simulink model "flow_control_while"  (R2013b)
settings: Solver=ode45  StartTime=0.0  StopTime=10.0  RelTol=1e-3
libraries: simulink x2
settings Model: Creator=Administrator  LastModifiedBy=Administrator

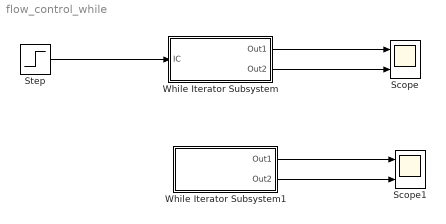
== system flow_control_while ==
  Scope : Scope  NumInputPorts=2
      settings: YMin=-5~-5  YMax=5~5
  Scope1 : Scope  NumInputPorts=2
      settings: YMin=-5~-5  YMax=5~5
  Step : Step  Time=5  SampleTime=0
  While Iterator Subsystem : Subsystem  TreatAsAtomicUnit=on
  While Iterator Subsystem1 : Subsystem  TreatAsAtomicUnit=on
  wires:
  Step/1 -> While Iterator Subsystem/1(IC)
  While Iterator Subsystem/1(Out1) -> Scope/1
  While Iterator Subsystem/2(Out2) -> Scope/2
  While Iterator Subsystem1/1(Out1) -> Scope1/1
  While Iterator Subsystem1/2(Out2) -> Scope1/2

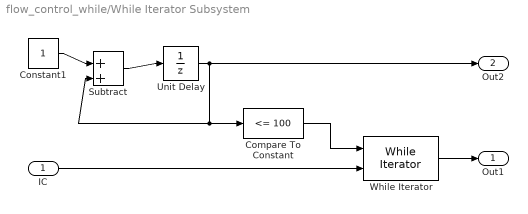
== system flow_control_while/While Iterator Subsystem ==
  IC : Inport
  Compare To Constant : simulink/Logic and Bit Operations/Compare To Constant  relop=<=  const=100  OutDataTypeStr=boolean
  Constant1 : Constant
  Subtract : Sum  Inputs=+|+
  Unit Delay : UnitDelay  SampleTime=-1
  While Iterator : WhileIterator  ShowIterationPort=on  OutputDataType=double
  Out1 : Outport
  Out2 : Outport  Port=2
  wires:
  IC/1 -> While Iterator/2
  While Iterator/1 -> Out1/1
  Constant1/1 -> Subtract/1
  Subtract/1 -> Unit Delay/1
  Unit Delay/1 -> Compare To Constant/1, Subtract/2, Out2/1
  Compare To Constant/1 -> While Iterator/1

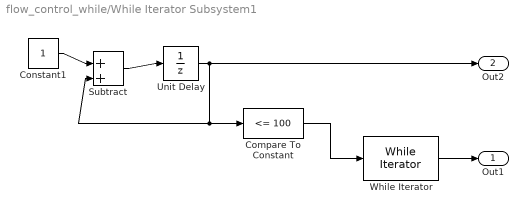
== system flow_control_while/While Iterator Subsystem1 ==
  Compare To Constant : simulink/Logic and Bit Operations/Compare To Constant  relop=<=  const=100  OutDataTypeStr=boolean
  Constant1 : Constant
  Subtract : Sum  Inputs=+|+
  Unit Delay : UnitDelay  SampleTime=-1
  While Iterator : WhileIterator  WhileBlockType=do-while  ShowIterationPort=on  OutputDataType=double
  Out1 : Outport
  Out2 : Outport  Port=2
  wires:
  While Iterator/1 -> Out1/1
  Constant1/1 -> Subtract/1
  Subtract/1 -> Unit Delay/1
  Unit Delay/1 -> Compare To Constant/1, Subtract/2, Out2/1
  Compare To Constant/1 -> While Iterator/1
